simulink model "MPU6050"  (R2013a)
settings: Solver=FixedStepDiscrete  SolverMode=SingleTasking  StartTime=0.0  StopTime=inf  FixedStep=0.03  RelTol=1e-3
undefined symbols (not defined in the file): DiscIntNeverNeededParam
libraries: arduinolib x6
settings Model: SimulationMode=external  ExtModeTrigDuration=2  Creator=Alec  LastModifiedBy=user
settings OptimizationCC: ExpressionDepthLimit=2147483647  OptimizeModelRefInitCode=on  LifeSpan=1
settings DebuggingCC: SolverPrmCheckMsg=none  StrictBusMsg=Warning
settings HardwareCC: ProdBitPerInt=16  ProdBitPerPointer=8  ProdIntDivRoundTo=Zero  ProdEndianess=LittleEndian  ProdWordSize=8  ProdHWDeviceType=Atmel->AVR
settings RTWCC: SystemTargetFile=realtime.tlc  GenerateMakefile=off  TemplateMakefile=realtime.tmf  Description=Real-Time Toolbox  RTWVerbose=off  ProcessScript=realtime_make_rtw_hook
settings CodeAppCC: CustomSymbolStrType=$N$R$M  InternalIdentifier=Classic
settings STFCustomTargetCC: TargetLibSuffix=.a  GenerateSampleERTMain=on  ERTCustomFileBanners=on  SupportNonInlinedSFcns=off  SupportVariableSizeSignals=on  MATLABClassNameForMDSCustomization=Simulink.SoftwareTarget.ERTCustomization  SystemTargetFile=realtime.tlc
settings ERTTargetCC: ParMdlRefBuildCompliant=off  CompOptLevelCompliant=off  ConcurrentExecutionCompliant=off  CombineOutputUpdateFcns=off  ERTFirstTimeCompliant=off  SupportContinuousTime=on  SupportVariableSizeSignals=on  ModelStepFunctionPrototypeControlCompliant=off  CPPClassGenCompliant=off  ExtMode=on  ExtModeTransport=3  ExtModeMexFile=ext_serial_win32_comm  ExtModeMexArgs=0 12 115200  ERTSrcFileBannerTemplate=realtime_code_template.cgt  ERTHdrFileBannerTemplate=realtime_code_template.cgt  ERTDataSrcFileTemplate=realtime_code_template.cgt  ERTDataHdrFileTemplate=realtime_code_template.cgt  ERTCustomFileTemplate=realtime_file_process.tlc

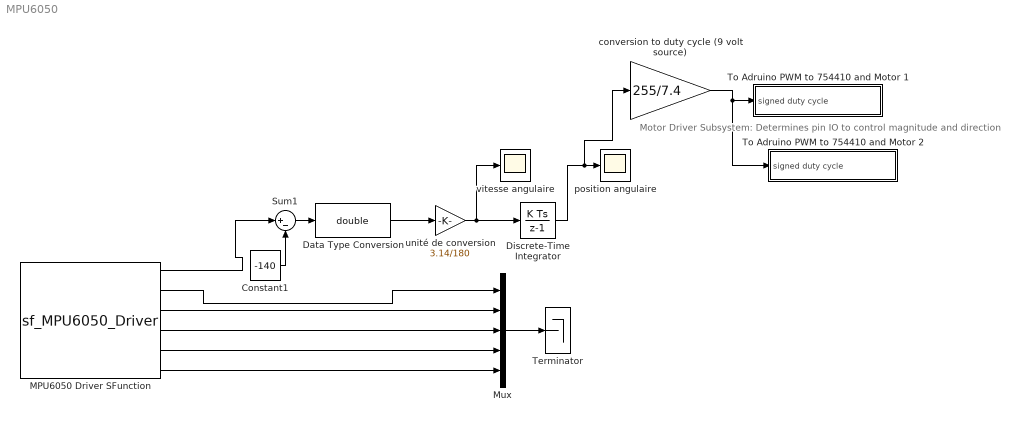
== system MPU6050 ==
  note: Motor Driver Subsystem:
      | Determines pin IO to control
      | magnitude and direction
  Constant1 : Constant  Value=-140
  Data Type Conversion : DataTypeConversion  OutDataTypeStr=double
  Discrete-Time Integrator : DiscreteIntegrator  SampleTime=0.03  ICPrevOutput=DiscIntNeverNeededParam  ICPrevScaledInput=DiscIntNeverNeededParam
  MPU6050 Driver SFunction : S-Function  InitFcn=try, set_param(gcb,'FunctionName','sf_MPU6050_Driver'), end  FunctionName=sf_MPU6050_Driver  SFunctionModules=sf_MPU6050_Driver_wrapper  EnableBusSupport=off  mask(S-Function Builder){}
      mask help: Simulink:masks:SFunctionBuilder_MD
      mask init:
      | val = [[.9  0.75 0.75 1 1 .9 .9 1]',[1 1 0.75 0.75 .9 .9 1 .9]'];try , sys = get_param(gcb,'SfunBuilderFcnName');if isempty(sys), sys = get_param(gcb,'FunctionName'); end,catch, sys = get_param(gcb,'FunctionName'); end
      settings: CopyFcn=set_param(gcbh,'LinkStatus','none')  PreSaveFcn=try, set_param(gcb,'FunctionName','sf_MPU6050_Driver'), end  OpenFcn=sfunctionwizard(gcbh)
      mask Display: plot(val(:,1),val(:,2)),disp(sys), port_label('output',1,'x_vel'), port_label('output',2,'y_vel'), port_label('output',3,'z_vel'), port_label('output',4,'x_acc'), port_label('output',5,'y_acc'), port_label('output',6,'z_acc')
  Mux : Mux  Inputs=5
  Sum1 : Sum  Inputs=|+-
  Terminator : Terminator
  To Adruino PWM to 754410 and Motor 1 : Subsystem
  To Adruino PWM to 754410 and Motor 2 : Subsystem
  conversion to duty cycle (9 volt source) : Gain  Gain=255/7.4
  position angulaire : Scope
      settings: TimeRange=10  YMin=17.5  YMax=60
  "unité de conversion " : Gain  Gain=3.14/180
  vitesse angulaire : Scope
      settings: TimeRange=10  YMin=-15  YMax=12.5
  wires:
  MPU6050 Driver SFunction/3 -> Mux/2
  MPU6050 Driver SFunction/6 -> Mux/5
  MPU6050 Driver SFunction/2 -> Mux/1
  MPU6050 Driver SFunction/5 -> Mux/4
  MPU6050 Driver SFunction/4 -> Mux/3
  Mux/1 -> Terminator/1
  MPU6050 Driver SFunction/1 -> Sum1/1
  Sum1/1 -> Data Type Conversion/1
  Constant1/1 -> Sum1/2
  Data Type Conversion/1 -> "unité de conversion "/1
  "unité de conversion "/1 -> vitesse angulaire/1, Discrete-Time Integrator/1
  Discrete-Time Integrator/1 -> conversion to duty cycle (9 volt source)/1, position angulaire/1
  conversion to duty cycle (9 volt source)/1 -> To Adruino PWM to 754410 and Motor 2/1(signed duty cycle), To Adruino PWM to 754410 and Motor 1/1(signed duty cycle)

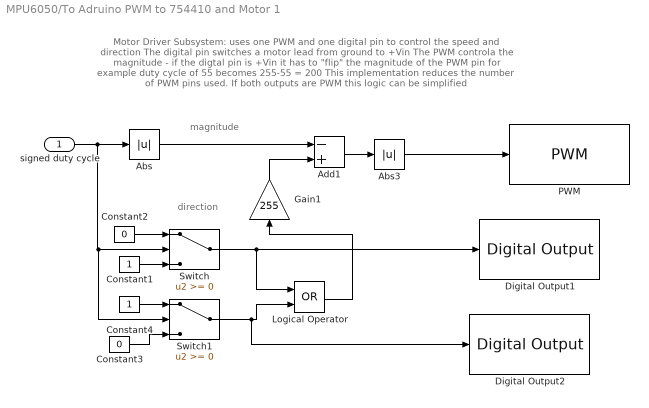
== system MPU6050/To Adruino PWM to 754410 and Motor 1 ==
  note: Motor Driver Subsystem: uses one PWM and one digital pin to control the speed and direction
      | The digital pin switches a motor lead from ground to +Vin
      | The PWM controla the magnitude - if the digtal pin is +Vin it has to "flip" the magnitude of the PWM pin
      | for example duty cycle of 55 becomes 255-55 = 200
      | This implementation reduces the number of PWM pins used.  If both outputs are PWM this logic can be simplified
  note: magnitude
  note: direction
  signed duty cycle : Inport
  Abs : Abs
  Abs3 : Abs
  Add1 : Sum  Inputs=-+
  Constant1 : Constant
  Constant2 : Constant  Value=0
  Constant3 : Constant  Value=0
  Constant4 : Constant
  Digital Output1 : arduinolib/Digital Output  pinNumber=4
  Digital Output2 : arduinolib/Digital Output  pinNumber=3
  Gain1 : Gain  Gain=255
  Logical Operator : Logic  Operator=OR  AllPortsSameDT=off  OutDataTypeStr=boolean
  PWM : arduinolib/PWM  pinNumber=9
  Switch : Switch
  Switch1 : Switch
  wires:
  signed duty cycle/1 -> Abs/1, Switch1/2, Switch/2
  Constant2/1 -> Switch/1
  Constant1/1 -> Switch/3
  Gain1/1 -> Add1/2
  Add1/1 -> Abs3/1
  Abs3/1 -> PWM/1
  Abs/1 -> Add1/1
  Switch/1 -> Digital Output1/1, Logical Operator/1
  Switch1/1 -> Digital Output2/1, Logical Operator/2
  Constant4/1 -> Switch1/1
  Constant3/1 -> Switch1/3
  Logical Operator/1 -> Gain1/1

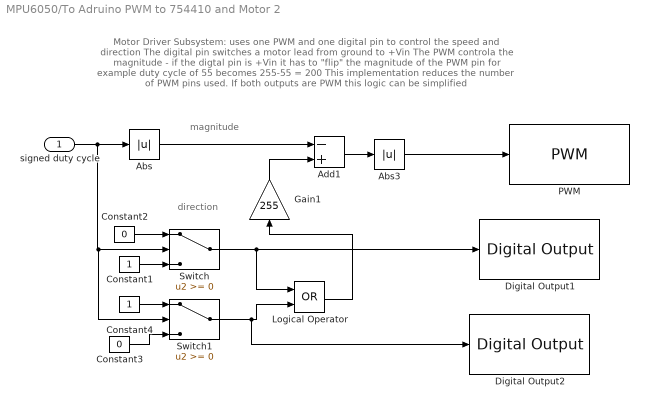
== system MPU6050/To Adruino PWM to 754410 and Motor 2 ==
  note: Motor Driver Subsystem: uses one PWM and one digital pin to control the speed and direction
      | The digital pin switches a motor lead from ground to +Vin
      | The PWM controla the magnitude - if the digtal pin is +Vin it has to "flip" the magnitude of the PWM pin
      | for example duty cycle of 55 becomes 255-55 = 200
      | This implementation reduces the number of PWM pins used.  If both outputs are PWM this logic can be simplified
  note: magnitude
  note: direction
  signed duty cycle : Inport
  Abs : Abs
  Abs3 : Abs
  Add1 : Sum  Inputs=-+
  Constant1 : Constant
  Constant2 : Constant  Value=0
  Constant3 : Constant  Value=0
  Constant4 : Constant
  Digital Output1 : arduinolib/Digital Output  pinNumber=7
  Digital Output2 : arduinolib/Digital Output  pinNumber=6
  Gain1 : Gain  Gain=255
  Logical Operator : Logic  Operator=OR  AllPortsSameDT=off  OutDataTypeStr=boolean
  PWM : arduinolib/PWM  pinNumber=10
  Switch : Switch
  Switch1 : Switch
  wires:
  signed duty cycle/1 -> Abs/1, Switch1/2, Switch/2
  Constant2/1 -> Switch/1
  Constant1/1 -> Switch/3
  Gain1/1 -> Add1/2
  Add1/1 -> Abs3/1
  Abs3/1 -> PWM/1
  Abs/1 -> Add1/1
  Switch/1 -> Digital Output1/1, Logical Operator/1
  Switch1/1 -> Digital Output2/1, Logical Operator/2
  Constant4/1 -> Switch1/1
  Constant3/1 -> Switch1/3
  Logical Operator/1 -> Gain1/1
